simulink model "task1"  (R2023a)
settings: Solver=VariableStepAuto  StartTime=0.0  StopTime=10.0  RelTol=1e-3
settings Model: Creator=user  LastModifiedBy=user

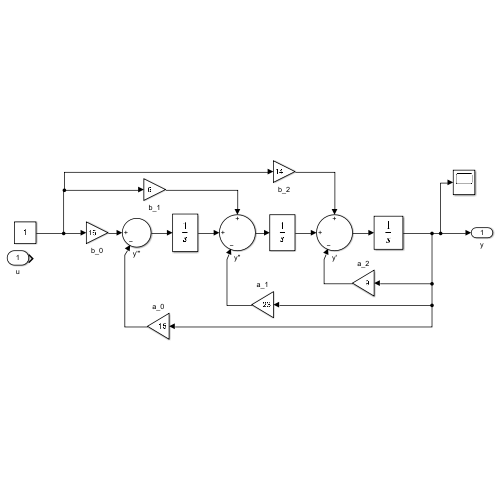
[thumbnail: Simulink's stored preview of the top-level diagram]
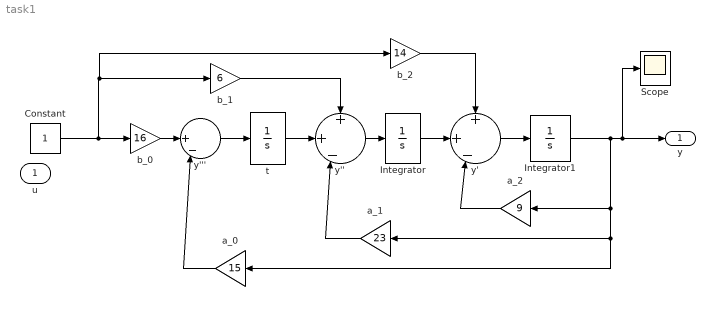
== system task1 ==
  u : Inport  OutMin=1  OutMax=1  Interpolate=off
  Constant : Constant
  Integrator : Integrator
  Integrator1 : Integrator
  Scope : Scope
  a_0 : Gain  Gain=15
  a_1 : Gain  Gain=23
  a_2 : Gain  Gain=9
  b_0 : Gain  Gain=16
  b_1 : Gain  Gain=6
  b_2 : Gain  Gain=14
  t : Integrator
  y' : Sum  Inputs=+|||+||-|
  y'' : Sum  Inputs=+|||+||-|
  y''' : Sum  Inputs=|||+|-|
  y : Outport
  wires:
  b_0/1 -> y'''/1
  y'''/1 -> t/1
  t/1 -> y''/2
  b_1/1 -> y''/1
  y''/1 -> Integrator/1
  Integrator/1 -> y'/2
  b_2/1 -> y'/1
  y'/1 -> Integrator1/1
  Integrator1/1 -> a_0/1, a_1/1, a_2/1, y/1, Scope/1
  a_0/1 -> y'''/2
  a_1/1 -> y''/3
  a_2/1 -> y'/3
  Constant/1 -> b_2/1, b_1/1, b_0/1
